simulink model "flo3_2018"  (R2018b)
settings: Solver=ode45  StartTime=0.0  StopTime=inf  FixedStep=0.01  RelTol=1e-3  EnableMultiTasking=on
settings Model: EnablePacing=on  Creator=Florian  LastModifiedBy=Florian
settings SolverCC: AutoInsertRateTranBlk=on
settings DataIOCC: LimitDataPoints=on  ReturnWorkspaceOutputs=on
settings OptimizationCC: LifeSpan=inf
settings DebuggingCC: AllowSymbolicDim=off  SFUnexpectedBacktrackingDiag=warning  SFNoUnconditionalDefaultTransitionDiag=warning  SFExecutionAtInitializationDiag=none  SFMachineParentedDataDiag=error
settings SFSimCC: SimUseLocalCustomCode=off
settings RTWCC: RTWUseLocalCustomCode=off
settings CodeAppCC: StateflowObjectComments=on
settings GRTTargetCC: TargetLangStandard=C89/C90 (ANSI)
settings ConfigComp: CovMetricSettings=dw  CovSaveCumulativeToWorkspaceVar=on  CovSaveSingleToWorkspaceVar=on  CovExternalEMLEnable=off  CovSFcnEnable=off

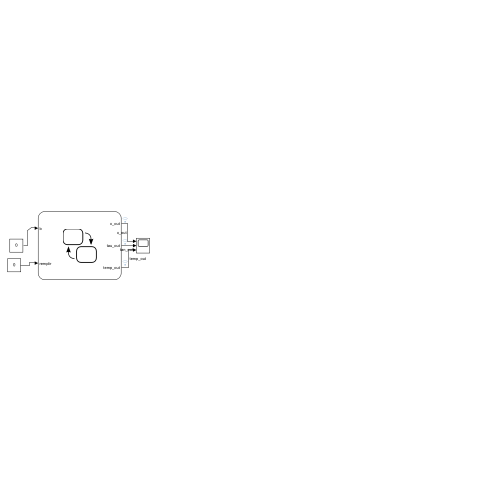
[thumbnail: Simulink's stored preview of the top-level diagram]
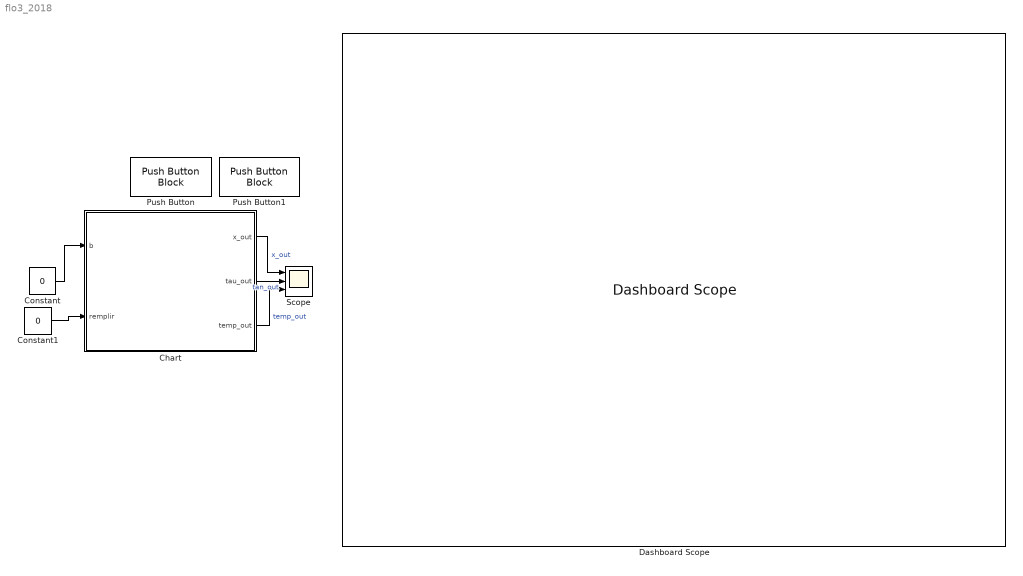
== system flo3_2018 ==
  Chart : Stateflow chart  TreatAsAtomicUnit=on
  Constant : Constant  Value=0
  Constant1 : Constant  Value=0
  Dashboard Scope : DashboardScope  Ymin=-1  Ymax=110  WebBlockId=7
  Push Button : PushButtonBlock  ButtonText=Café  OffValue=0.000000  WebBlockId=15
  Push Button1 : PushButtonBlock  ButtonText=Remplir  OffValue=0.000000  WebBlockId=16
  Scope : Scope  NumInputPorts=3
  wires:
  Chart/1(x_out) -> Scope/1  "x_out"
  Chart/2(tau_out) -> Scope/2  "tan_out"
  Constant/1 -> Chart/1(b)
  Constant1/1 -> Chart/2(remplir)
  Chart/3(temp_out) -> Scope/3  "temp_out"

== stateflow chart flo3_2018/Chart ==
  settings: updateMethod=CONTINUOUS  executeAtInitialization=1  initializeOutput=1
  state Q0
    du:
    %derivative
    x_dot=0;
    tau_dot=0;
    temp_dot = -(perte*(x_max-x)+cst);
    %output
    x_out = x;
    tau_out = tau;
    temp_out = temp;
  state Q1
    du:
    %derivative
    x_dot=-alpha;
    tau_dot=1;
    temp_dot = -(perte*(x_max-x)+cst);
    %output
    x_out = x;
    tau_out = tau;
    temp_out = temp;
  state Q02
    du:
    %derivative
    x_dot=0;
    tau_dot=0;
    temp_dot=chauffe*x + cst;
    %output
    x_out = x;
    tau_out = tau;
    temp_out = temp;
  state Q03
    du:
    %derivative
    x_dot=0;
    tau_dot=0;
    temp_dot=chauffe*x+cst;
    %output
    x_out = x;
    tau_out = tau;
    temp_out = temp;
  (default) -> Q0 : {x =100
      | tau = 0
      | temp = 0}
  Q0 -> Q0 [order 3] : [x <= x_min && remplir]{x = x_max}
  Q0 -> Q1 [order 1] : [b && x > x_min && temp > 70]{tau = 0}
  Q1 -> Q0 : [tau >= tau_max || x <= 0]
  Q0 -> Q02 [order 2] : [temp <= 70 && x > x_min]
  Q02 -> Q0 [order 1] : [temp >= 80]
  Q03 -> Q1 : [temp >= 75]{tau = 0}
  Q02 -> Q03 [order 2] : [b && x > x_min && temp < 80]
  data: x local double; tau local double; x_out output double size=1; tau_out output double size=1; tau_max constant double =4; alpha constant double =3; b input; x_max local =100; remplir input; temp local; temp_out output; perte constant double =0.002; chauffe constant double =0.01; cst constant double =1; x_min local =10
  data x settings: updateMethod=SF_CONTINUOUS_TIME_DATA
  data tau settings: updateMethod=SF_CONTINUOUS_TIME_DATA
  data x_max settings: updateMethod=SF_CONTINUOUS_TIME_DATA
  data temp settings: updateMethod=SF_CONTINUOUS_TIME_DATA
  data x_min settings: updateMethod=SF_CONTINUOUS_TIME_DATA
